simulink model "LLC_modulator_analysis"  (R2025b)
settings: Solver=VariableStepAuto  StartTime=0.0  StopTime=0.0005  RelTol=1e-3
undefined symbols (not defined in the file): fPWM_DAB, fPWM_LLC_pu, fres
libraries: resonant_llc_modulator x1
settings Model: Creator=ltnbda  LastModifiedBy=dbagn

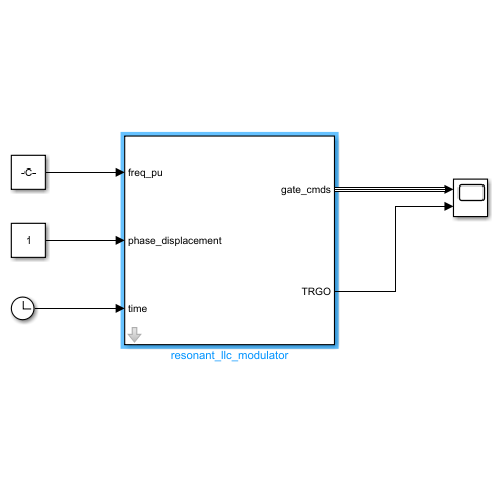
[thumbnail: Simulink's stored preview of the top-level diagram]
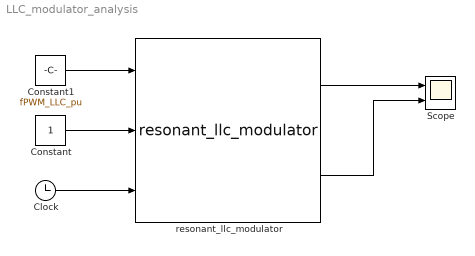
== system LLC_modulator_analysis ==
  Clock : Clock
  Constant : Constant
  Constant1 : Constant  Value=fPWM_LLC_pu
  Scope : Scope  NumInputPorts=2
      settings: ActiveDisplayYMinimum=-13.125  ActiveDisplayYMaximum=18.125
  resonant_llc_modulator : resonant_llc_modulator/resonant_llc_modulator  freq_base=fPWM_DAB  fres=fres*1.5  pos_cmd_gate=15  neg_cmd_gate=-10  tc=500e-9  trgo_double_update=0  max_phase_displacement=pi/2  freq_min=fPWM_DAB/5  freq_max=fPWM_DAB*0.625
  wires:
  Clock/1 -> resonant_llc_modulator/3
  Constant/1 -> resonant_llc_modulator/2
  Constant1/1 -> resonant_llc_modulator/1
  resonant_llc_modulator/1 -> Scope/1
  resonant_llc_modulator/2 -> Scope/2
